simulink model "homework_2_sim_local_obs"  (R2018b)
settings: Solver=VariableStepAuto  StartTime=0.0  StopTime=15  MaxStep=1e-2  MinStep=1e-3  RelTol=1e-3
values from neighbouring files (symbols this model uses):
  A = A-B*K0    [homework_2_dist_obs.m]    (also in homework_2_local_obs.m)
  B = [0 -9.9453]'    [homework_2_dist_obs.m]    (also in homework_2_local_obs.m)
  c = 10*1/(2*min(real(lam_g)))    [homework_2_dist_obs.m]    (also in homework_2_local_obs.m = 5*1/(2*min(real(lam_g))))
  C = [708.27 0]    [homework_2_dist_obs.m]    (also in homework_2_local_obs.m)
  D = [0]    [homework_2_dist_obs.m]    (also in homework_2_local_obs.m)
  F = P*C'*R^-1    [homework_2_dist_obs.m]    (also in homework_2_local_obs.m = place(A', -c*C', [-10; -20])')
  G_ext = zeros(7, 7)    [homework_2_dist_obs.m]    (also in homework_2_local_obs.m)
  K = R^-1*B'*P    [homework_2_dist_obs.m]    (also in homework_2_local_obs.m)
  x0_f = [0.1818 0.1455; 0.8693 0.5499; 0.8530 0.3510;      0.2638 0.1361; 0.5797 0.1450; 0.6221 0.5132]'    [homework_2_dist_obs.m]    (also in homework_2_local_obs.m)
  x0_l = [1 1]    [homework_2_dist_obs.m]    (also in homework_2_local_obs.m)
libraries: simulink x6
settings Model: Creator=esmer  LastModifiedBy=mluser
settings DataIOCC: ReturnWorkspaceOutputs=on

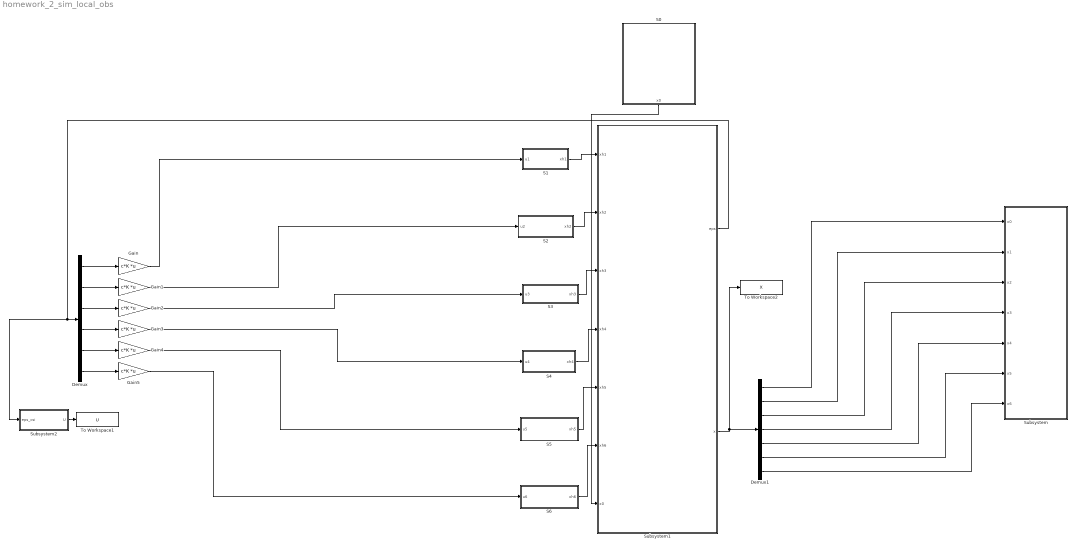
== system homework_2_sim_local_obs ==
  Demux : Demux  Outputs=6
  Demux1 : Demux  Outputs=7
  Gain{,1..5} (6 alike) : Gain  Gain=c*K  Multiplication=Matrix(K*u)
  S0 : Subsystem
  S1 : Subsystem
  S2 : Subsystem
  S3 : Subsystem
  S4 : Subsystem
  S5 : Subsystem
  S6 : Subsystem
  Subsystem : Subsystem
  Subsystem1 : Subsystem
  Subsystem2 : Subsystem
  To Workspace1 : ToWorkspace  VariableName=U  SaveFormat=Timeseries  SampleTime=-1
  To Workspace2 : ToWorkspace  VariableName=X  SaveFormat=Timeseries  SampleTime=-1
  wires:
  Subsystem1/1(eps) -> Subsystem2/1(eps_csi), Demux/1
  Demux/1 -> Gain/1
  Demux/2 -> Gain1/1
  Demux/3 -> Gain2/1
  Demux/4 -> Gain3/1
  Demux/5 -> Gain4/1
  Demux/6 -> Gain5/1
  Gain1/1 -> S2/1(u2)
  Gain2/1 -> S3/1(u3)
  Gain3/1 -> S4/1(u4)
  Gain4/1 -> S5/1(u5)
  Gain5/1 -> S6/1(u6)
  S0/1(x0) -> Subsystem1/7(x0)
  S1/1(xh1) -> Subsystem1/1(xh1)
  S2/1(xh2) -> Subsystem1/2(xh2)
  S3/1(xh3) -> Subsystem1/3(xh3)
  S4/1(xh4) -> Subsystem1/4(xh4)
  S5/1(xh5) -> Subsystem1/5(xh5)
  S6/1(xh6) -> Subsystem1/6(xh6)
  Subsystem1/2(x) -> Demux1/1, To Workspace2/1
  Demux1/1 -> Subsystem/1(x0)
  Demux1/2 -> Subsystem/2(x1)
  Demux1/3 -> Subsystem/3(x2)
  Demux1/4 -> Subsystem/4(x3)
  Demux1/5 -> Subsystem/5(x4)
  Demux1/6 -> Subsystem/6(x5)
  Demux1/7 -> Subsystem/7(x6)
  Gain/1 -> S1/1(u1)
  Subsystem2/1(U) -> To Workspace1/1

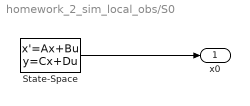
== system homework_2_sim_local_obs/S0 ==
  State-Space : StateSpace  A=A  B=B  C=eye(2)  D=zeros(2,1)  InitialCondition=x0_l
  x0 : Outport
  wires:
  State-Space/1 -> x0/1

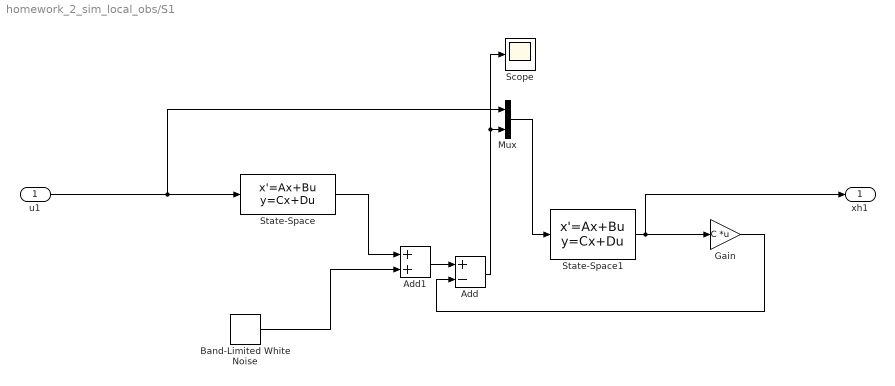
== system homework_2_sim_local_obs/S1 ==
  u1 : Inport
  Add : Sum  Inputs=+-
  Add1 : Sum
  Band-Limited White Noise : simulink/Sources/Band-Limited White Noise  Cov=n  Ts=0.1  seed=[23341]
  Gain : Gain  Gain=C  Multiplication=Matrix(K*u)
  Mux : Mux  Inputs=2
  Scope : Scope
  State-Space : StateSpace  A=A  B=B  C=C  D=D  InitialCondition=x0_f(:,1)
  State-Space1 : StateSpace  A=A  B=[B -c*F]  C=eye(2)  D=[zeros(2, 1) zeros(2,1)]  InitialCondition=0
  xh1 : Outport
  wires:
  u1/1 -> Mux/1, State-Space/1
  Add/1 -> Scope/1, Mux/2
  Mux/1 -> State-Space1/1
  Gain/1 -> Add/2
  State-Space1/1 -> xh1/1, Gain/1
  Add1/1 -> Add/1
  State-Space/1 -> Add1/1
  Band-Limited White Noise/1 -> Add1/2

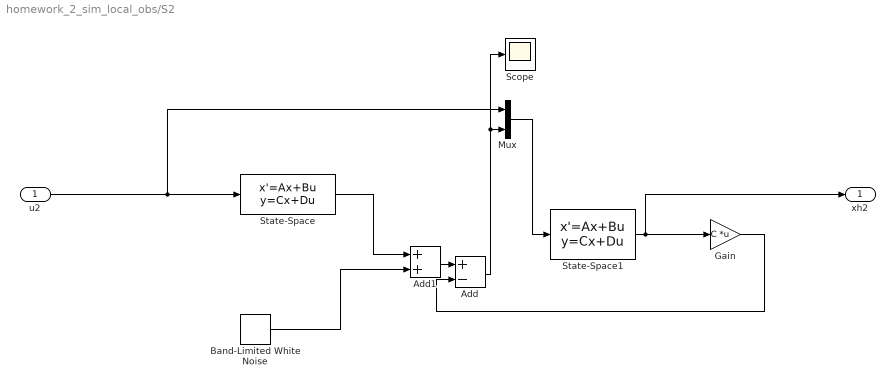
== system homework_2_sim_local_obs/S2 ==
  u2 : Inport
  Add : Sum  Inputs=+-
  Add1 : Sum
  Band-Limited White Noise : simulink/Sources/Band-Limited White Noise  Cov=n  Ts=0.1  seed=[23441]
  Gain : Gain  Gain=C  Multiplication=Matrix(K*u)
  Mux : Mux  Inputs=2
  Scope : Scope
  State-Space : StateSpace  A=A  B=B  C=C  D=D  InitialCondition=x0_f(:,2)
  State-Space1 : StateSpace  A=A  B=[B -c*F]  C=eye(2)  D=[zeros(2, 1) zeros(2,1)]  InitialCondition=0
  xh2 : Outport
  wires:
  Mux/1 -> State-Space1/1
  Gain/1 -> Add/2
  Add/1 -> Scope/1, Mux/2
  State-Space1/1 -> xh2/1, Gain/1
  u2/1 -> Mux/1, State-Space/1
  Add1/1 -> Add/1
  State-Space/1 -> Add1/1
  Band-Limited White Noise/1 -> Add1/2

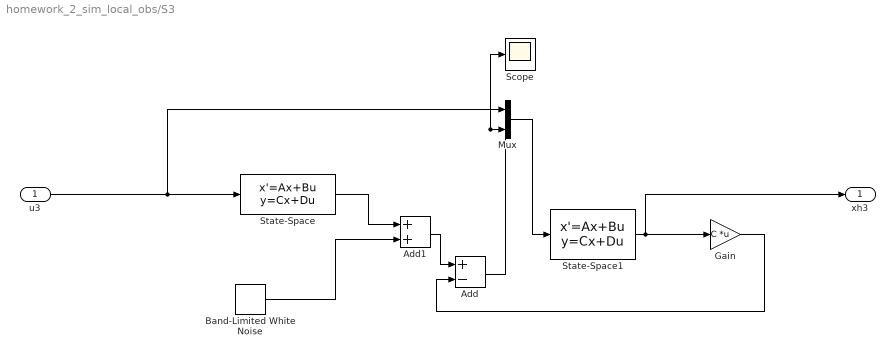
== system homework_2_sim_local_obs/S3 ==
  u3 : Inport
  Add : Sum  Inputs=+-
  Add1 : Sum
  Band-Limited White Noise : simulink/Sources/Band-Limited White Noise  Cov=n  Ts=0.1  seed=[23541]
  Gain : Gain  Gain=C  Multiplication=Matrix(K*u)
  Mux : Mux  Inputs=2
  Scope : Scope
  State-Space : StateSpace  A=A  B=B  C=C  D=D  InitialCondition=x0_f(:,3)
  State-Space1 : StateSpace  A=A  B=[B -c*F]  C=eye(2)  D=[zeros(2, 1) zeros(2,1)]  InitialCondition=0
  xh3 : Outport
  wires:
  Mux/1 -> State-Space1/1
  Gain/1 -> Add/2
  Add/1 -> Scope/1, Mux/2
  State-Space1/1 -> xh3/1, Gain/1
  u3/1 -> Mux/1, State-Space/1
  Add1/1 -> Add/1
  State-Space/1 -> Add1/1
  Band-Limited White Noise/1 -> Add1/2

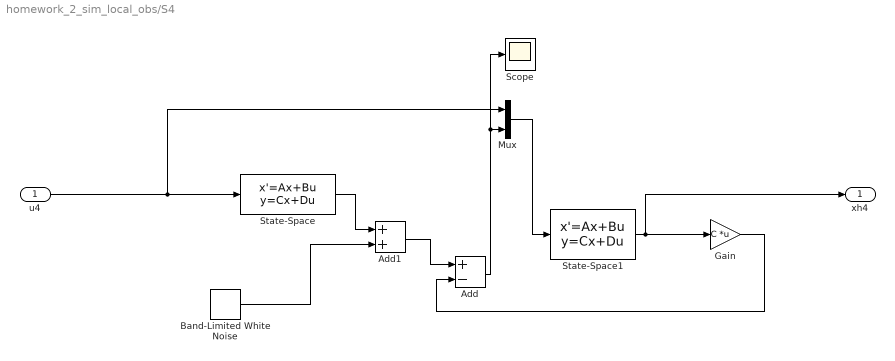
== system homework_2_sim_local_obs/S4 ==
  u4 : Inport
  Add : Sum  Inputs=+-
  Add1 : Sum
  Band-Limited White Noise : simulink/Sources/Band-Limited White Noise  Cov=n  Ts=0.1  seed=[23641]
  Gain : Gain  Gain=C  Multiplication=Matrix(K*u)
  Mux : Mux  Inputs=2
  Scope : Scope
  State-Space : StateSpace  A=A  B=B  C=C  D=D  InitialCondition=x0_f(:,4)
  State-Space1 : StateSpace  A=A  B=[B -c*F]  C=eye(2)  D=[zeros(2, 1) zeros(2,1)]  InitialCondition=0
  xh4 : Outport
  wires:
  Mux/1 -> State-Space1/1
  Gain/1 -> Add/2
  Add/1 -> Scope/1, Mux/2
  State-Space1/1 -> xh4/1, Gain/1
  u4/1 -> Mux/1, State-Space/1
  Add1/1 -> Add/1
  State-Space/1 -> Add1/1
  Band-Limited White Noise/1 -> Add1/2

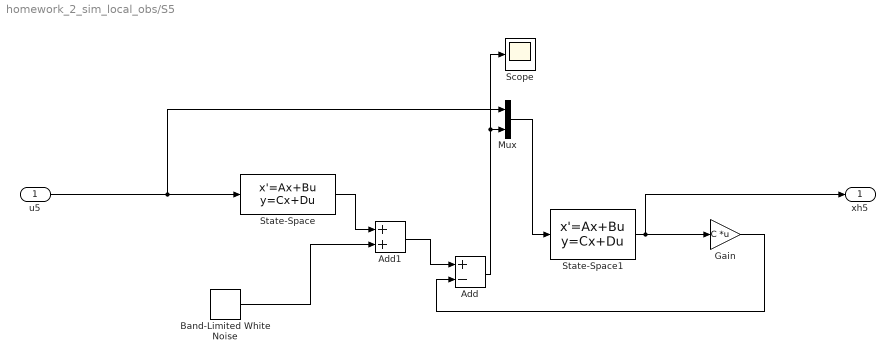
== system homework_2_sim_local_obs/S5 ==
  u5 : Inport
  Add : Sum  Inputs=+-
  Add1 : Sum
  Band-Limited White Noise : simulink/Sources/Band-Limited White Noise  Cov=n  Ts=0.1  seed=[23741]
  Gain : Gain  Gain=C  Multiplication=Matrix(K*u)
  Mux : Mux  Inputs=2
  Scope : Scope
  State-Space : StateSpace  A=A  B=B  C=C  D=D  InitialCondition=x0_f(:,5)
  State-Space1 : StateSpace  A=A  B=[B -c*F]  C=eye(2)  D=[zeros(2, 1) zeros(2,1)]  InitialCondition=0
  xh5 : Outport
  wires:
  Mux/1 -> State-Space1/1
  Gain/1 -> Add/2
  Add/1 -> Scope/1, Mux/2
  State-Space1/1 -> xh5/1, Gain/1
  u5/1 -> Mux/1, State-Space/1
  Add1/1 -> Add/1
  State-Space/1 -> Add1/1
  Band-Limited White Noise/1 -> Add1/2

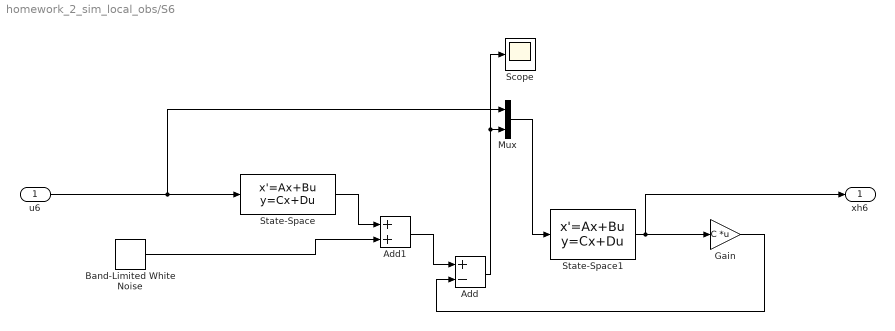
== system homework_2_sim_local_obs/S6 ==
  u6 : Inport
  Add : Sum  Inputs=+-
  Add1 : Sum
  Band-Limited White Noise : simulink/Sources/Band-Limited White Noise  Cov=n  Ts=0.1  seed=[23841]
  Gain : Gain  Gain=C  Multiplication=Matrix(K*u)
  Mux : Mux  Inputs=2
  Scope : Scope
  State-Space : StateSpace  A=A  B=B  C=C  D=D  InitialCondition=x0_f(:,6)
  State-Space1 : StateSpace  A=A  B=[B -c*F]  C=eye(2)  D=[zeros(2, 1) zeros(2,1)]  InitialCondition=0
  xh6 : Outport
  wires:
  Mux/1 -> State-Space1/1
  Gain/1 -> Add/2
  Add/1 -> Scope/1, Mux/2
  State-Space1/1 -> xh6/1, Gain/1
  u6/1 -> Mux/1, State-Space/1
  Add1/1 -> Add/1
  State-Space/1 -> Add1/1
  Band-Limited White Noise/1 -> Add1/2

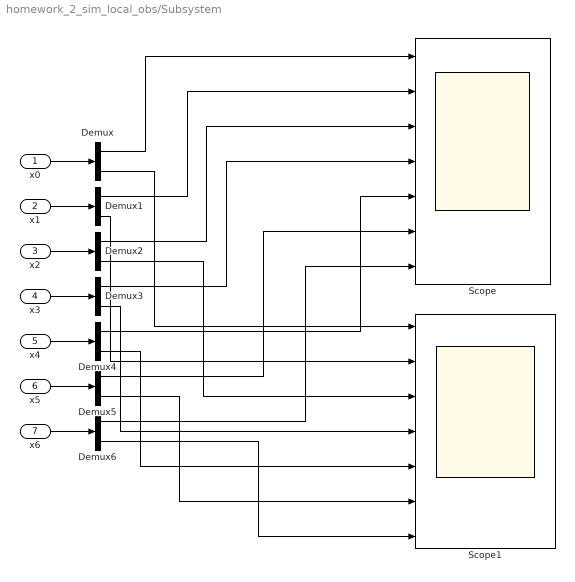
== system homework_2_sim_local_obs/Subsystem ==
  x0 : Inport
  x1 : Inport  Port=2
  x2 : Inport  Port=3
  x3 : Inport  Port=4
  x4 : Inport  Port=5
  x5 : Inport  Port=6
  x6 : Inport  Port=7
  Demux{,1..6} (7 alike) : Demux  Outputs=2
  Scope : Scope  NumInputPorts=7
  Scope1 : Scope  NumInputPorts=7
  wires:
  x0/1 -> Demux/1
  x6/1 -> Demux6/1
  x5/1 -> Demux5/1
  x4/1 -> Demux4/1
  x3/1 -> Demux3/1
  x2/1 -> Demux2/1
  x1/1 -> Demux1/1
  Demux/1 -> Scope/1
  Demux1/1 -> Scope/2
  Demux2/1 -> Scope/3
  Demux3/1 -> Scope/4
  Demux5/1 -> Scope/6
  Demux6/1 -> Scope/7
  Demux/2 -> Scope1/1
  Demux1/2 -> Scope1/2
  Demux2/2 -> Scope1/3
  Demux4/1 -> Scope/5
  Demux3/2 -> Scope1/4
  Demux4/2 -> Scope1/5
  Demux5/2 -> Scope1/6
  Demux6/2 -> Scope1/7

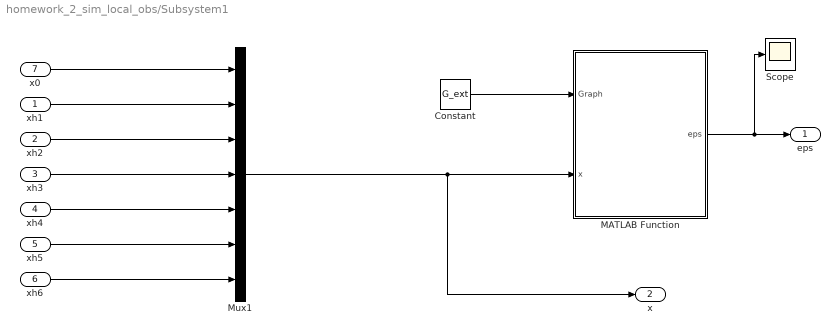
== system homework_2_sim_local_obs/Subsystem1 ==
  xh1 : Inport
  xh2 : Inport  Port=2
  xh3 : Inport  Port=3
  xh4 : Inport  Port=4
  xh5 : Inport  Port=5
  xh6 : Inport  Port=6
  x0 : Inport  Port=7
  Constant : Constant  Value=G_ext
  MATLAB Function : MATLAB Function  TreatAsAtomicUnit=on
  Mux1 : Mux  Inputs=7
  Scope : Scope
  eps : Outport
  x : Outport  Port=2
  wires:
  Mux1/1 -> x/1, MATLAB Function/2(x)
  Constant/1 -> MATLAB Function/1(Graph)
  MATLAB Function/1(eps) -> Scope/1, eps/1
  xh6/1 -> Mux1/7
  xh5/1 -> Mux1/6
  xh4/1 -> Mux1/5
  xh3/1 -> Mux1/4
  xh2/1 -> Mux1/3
  xh1/1 -> Mux1/2
  x0/1 -> Mux1/1

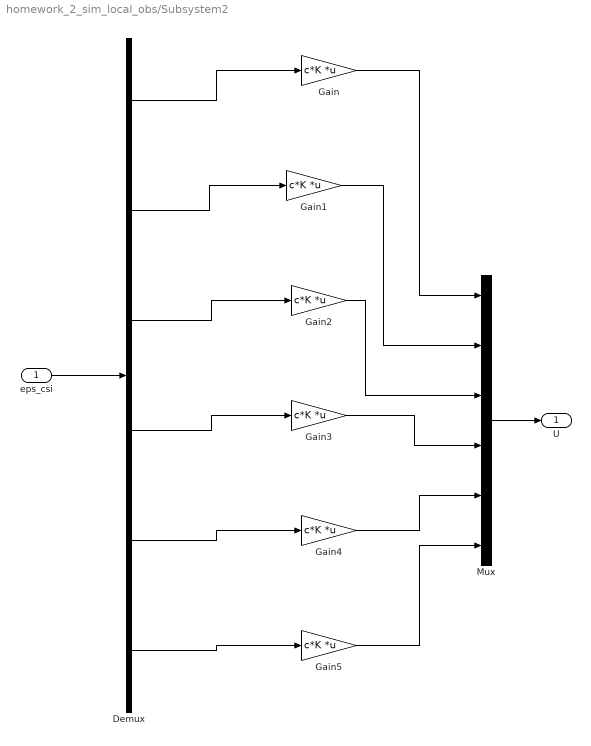
== system homework_2_sim_local_obs/Subsystem2 ==
  eps_csi : Inport
  Demux : Demux  Outputs=6
  Gain{,1..5} (6 alike) : Gain  Gain=c*K  Multiplication=Matrix(K*u)
  Mux : Mux  Inputs=6
  U : Outport
  wires:
  eps_csi/1 -> Demux/1
  Mux/1 -> U/1
  Gain/1 -> Mux/1
  Gain1/1 -> Mux/2
  Gain2/1 -> Mux/3
  Gain3/1 -> Mux/4
  Gain4/1 -> Mux/5
  Gain5/1 -> Mux/6
  Demux/1 -> Gain/1
  Demux/2 -> Gain1/1
  Demux/3 -> Gain2/1
  Demux/4 -> Gain3/1
  Demux/5 -> Gain4/1
  Demux/6 -> Gain5/1

== matlab function homework_2_sim_local_obs/Subsystem1/MATLAB Function ==
  data: Graph input; eps output; x input
function eps = fcn(Graph, x)

tmp = zeros(2, 6);
x0=x(1:2);
x=reshape(x(3:end), 2, 6);
Adj=Graph(2:end, 2:end);
G=Graph(2:end,1);
for i=1:6 %calcolo eps per ogni nodo
    tmp(:,i) = G(i)*(x0-x(:,i));
    %contributo altri nodi
    for j = 1:6 
        tmp(:,i) = tmp(:,i) + Adj(i, j)*(x(:,j)-x(:,i));
    end
end
eps=reshape(tmp, 12, 1);
end
